simulink model "test"  (R2021b)
settings: Solver=FixedStepDiscrete  StartTime=0.0  StopTime=0.2  FixedStep=1e-6  RelTol=1e-3
InitFcn:
  | init_fcn
values from neighbouring files (symbols this model uses):
  Tint = 1e-6    (= 1e-06)    [init_fcn.m]
libraries: spsIGBTDiodeLib x6, spsVoltageMeasurementLib x4, spsSeriesRLCBranchLib x4, spsCurrentMeasurementLib x3, simulink x1, spsThreePhaseSourceLib x1, spspowerguiLib x1
settings Model: Creator=david  LastModifiedBy=david

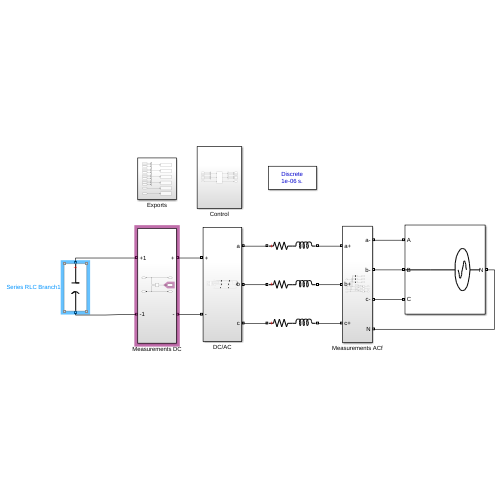
[thumbnail: Simulink's stored preview of the top-level diagram]
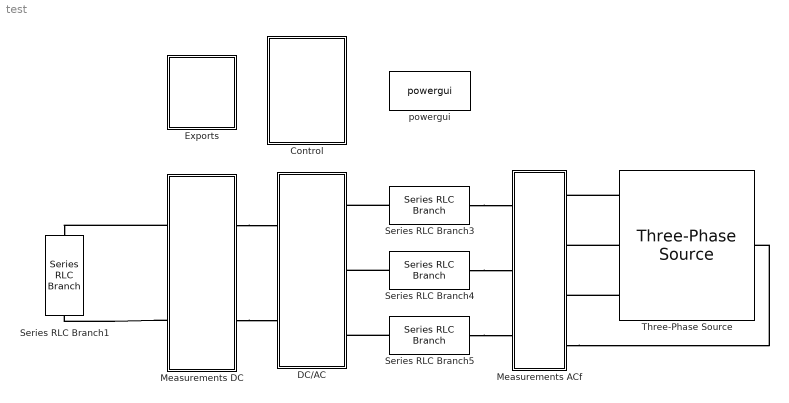
== system test ==
  Control : Subsystem
  DC/AC : Subsystem
  Exports : Subsystem
  Measurements ACf : Subsystem
  Measurements DC : Subsystem
  Series RLC Branch1 : spsSeriesRLCBranchLib/Series RLC Branch  LConnTagsString=__new0  RConnTagsString=__new0  BranchType=C  Resistance=0.2  Inductance=5e-3  SetiL0=off  InitialCurrent=0  Capacitance=3300e-6  Setx0=on  InitialVoltage=560  Measurements=None
  Series RLC Branch3 : spsSeriesRLCBranchLib/Series RLC Branch  LConnTagsString=__new0  RConnTagsString=__new0  BranchType=RL  Resistance=0.2  Inductance=5e-3  SetiL0=off  InitialCurrent=0  Capacitance=0  Setx0=off  InitialVoltage=0  Measurements=None
  Series RLC Branch4 : spsSeriesRLCBranchLib/Series RLC Branch  LConnTagsString=__new0  RConnTagsString=__new0  BranchType=RL  Resistance=0.2  Inductance=5e-3  SetiL0=off  InitialCurrent=0  Capacitance=0  Setx0=off  InitialVoltage=0  Measurements=None
  Series RLC Branch5 : spsSeriesRLCBranchLib/Series RLC Branch  LConnTagsString=__new0  RConnTagsString=__new0  BranchType=RL  Resistance=0.2  Inductance=5e-3  SetiL0=off  InitialCurrent=0  Capacitance=0  Setx0=off  InitialVoltage=0  Measurements=None
  Three-Phase Source : spsThreePhaseSourceLib/Three-Phase Source  InternalConnection=Yn  VoltagePhases=off  Voltage=400  PhaseAngle=0  Voltage_phases=[25e3 25e3 25e3]/sqrt(3)  PhaseAngles_phases=[0 -120 +120]  Frequency=50  NonIdealSource=on  SpecifyImpedance=off  Resistance=0  Inductance=0  ShortCircuitLevel=100e6  BaseVoltage=400  XRratio=7  BusType=swing  Pref=10e3  Qref=0  Prefabc=[10e3, 10e3, 10e3]  Qrefabc=[0, 0, 0]  Qmin=-inf  Qmax=inf
  powergui : spspowerguiLib/powergui  Priority=1  SimulationMode=Discrete  SampleTime=Tint  frequency=60  Iterations=50  frequencyindice=0  Pbase=100e6  ErrMax=1e-4  UnitsV=kV  UnitsW=MW  buscounter=0  FunctionMessages=off  echomessages=off  EnableUseOfTLC=off  CurrentSourceSwitches=off  DisableSnubberDevices=off  DisableRonSwitches=off  DisableVfSwitches=off  DisplayEquations=off  AutomaticDiscreteSolvers=off  SolverType=Tustin/Backward Euler (TBE)  Interpol=off  ExternalGateDelay=off  methode=off  Ts=100  x0status=blocks  SPID=on  SwTol=0  HookPort=off  NonlinearTolerance=1e-4  nMaxIteration=100  ContinueOnMaxIteration=off  RestoreLinks=warning  ResistiveCurrentMeasurement=off  Frange=[0:2:500]  Ylog=off  Xlog=on  ShowGrid=off  save=off  variable=ZData  structure=0  ZoomFFT=off  StartTime=0.0  cycles=1  DisplayStyle=1  fundamental=60  FreqAxis=off  MaxFrequency=1000  frequencyindicesteady=1  RmsSteady=1  display=off
  connections:
  Series RLC Branch3/LConn1 -- DC/AC/RConn1
  Measurements DC/LConn2 -- Series RLC Branch1/RConn1
  Measurements DC/LConn1 -- Series RLC Branch1/LConn1
  Measurements DC/RConn1 -- DC/AC/LConn1
  Measurements DC/RConn2 -- DC/AC/LConn2
  Series RLC Branch5/LConn1 -- DC/AC/RConn3
  Series RLC Branch4/LConn1 -- DC/AC/RConn2
  Three-Phase Source/RConn1 -- Measurements ACf/RConn1
  Three-Phase Source/RConn2 -- Measurements ACf/RConn2
  Three-Phase Source/RConn3 -- Measurements ACf/RConn3
  Series RLC Branch3/RConn1 -- Measurements ACf/LConn1
  Series RLC Branch5/RConn1 -- Measurements ACf/LConn3
  Series RLC Branch4/RConn1 -- Measurements ACf/LConn2
  Measurements ACf/RConn4 -- Three-Phase Source/LConn1

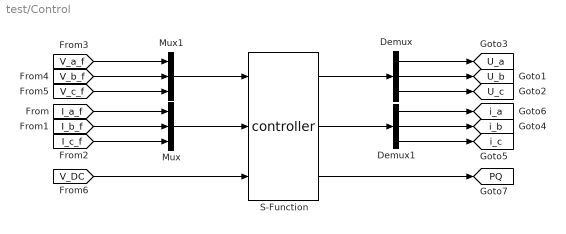
== system test/Control ==
  Demux : Demux  Outputs=3
  Demux1 : Demux  Outputs=3
  Mux : Mux  Inputs=3
  Mux1 : Mux  Inputs=3
  S-Function : S-Function  FunctionName=controller  SFunctionDeploymentMode=off  EnableBusSupport=off
  tag scope: PQ=global, U_a=global, U_b=global, U_c=global, i_a=global, i_b=global, i_c=global
  wires:
  [I_a_f] -> Mux/1
  [I_c_f] -> Mux/3
  Mux1/1 -> S-Function/1
  [V_a_f] -> Mux1/1
  [V_c_f] -> Mux1/3
  [I_b_f] -> Mux/2
  [V_b_f] -> Mux1/2
  Mux/1 -> S-Function/2
  S-Function/1 -> Demux/1
  S-Function/2 -> Demux1/1
  Demux/1 -> [U_a]
  Demux/2 -> [U_b]
  Demux/3 -> [U_c]
  Demux1/1 -> [i_a]
  Demux1/2 -> [i_b]
  Demux1/3 -> [i_c]
  S-Function/3 -> [PQ]
  [V_DC] -> S-Function/3

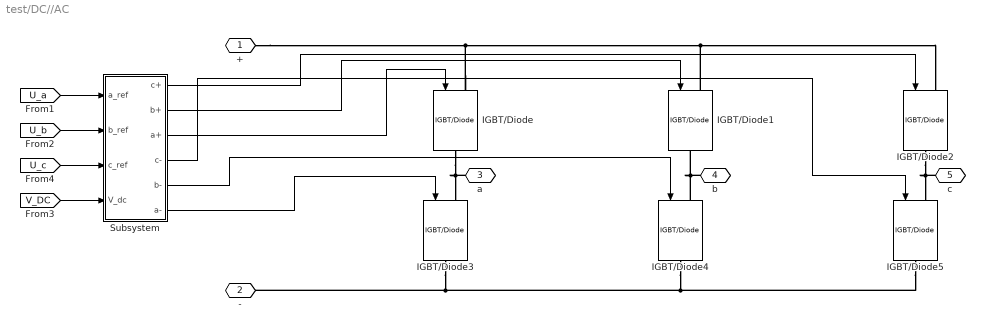
== system test/DC//AC ==
  IGBT/Diode{,1..5} (6 alike) : spsIGBTDiodeLib/IGBT//Diode  Ron=1e-3  Rs=1e5  Cs=inf  Measurements=off
  Subsystem : Subsystem
  + : PMIOPort  Side=Left
  - : PMIOPort  Port=2  Side=Left
  a : PMIOPort  Port=3  Side=Right
  b : PMIOPort  Port=4  Side=Right
  c : PMIOPort  Port=5  Side=Right
  wires:
  Subsystem/3(a+) -> IGBT/Diode/1
  Subsystem/2(b+) -> IGBT/Diode1/1
  Subsystem/5(b-) -> IGBT/Diode4/1
  Subsystem/1(c+) -> IGBT/Diode2/1
  Subsystem/4(c-) -> IGBT/Diode5/1
  [V_DC] -> Subsystem/4(V_dc)
  Subsystem/6(a-) -> IGBT/Diode3/1
  [U_b] -> Subsystem/2(b_ref)
  [U_c] -> Subsystem/3(c_ref)
  [U_a] -> Subsystem/1(a_ref)
  connections:
  IGBT/Diode2/RConn1 -- c/RConn1 -- IGBT/Diode5/LConn1
  IGBT/Diode/RConn1 -- a/RConn1 -- IGBT/Diode3/LConn1
  IGBT/Diode4/LConn1 -- b/RConn1 -- IGBT/Diode1/RConn1
  IGBT/Diode5/RConn1 -- IGBT/Diode4/RConn1 -- IGBT/Diode3/RConn1 -- -/RConn1
  IGBT/Diode/LConn1 -- IGBT/Diode2/LConn1 -- IGBT/Diode1/LConn1 -- +/RConn1

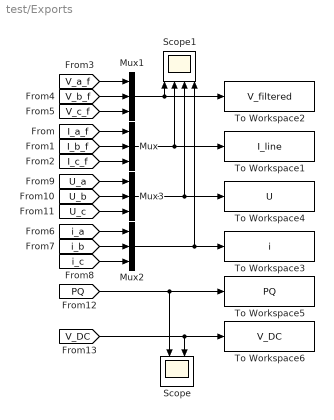
== system test/Exports ==
  Mux{,1..3} (4 alike) : Mux  Inputs=3
  Scope : Scope  NumInputPorts=2
  Scope1 : Scope  NumInputPorts=4
  To Workspace1 : ToWorkspace  VariableName=I_line  SaveFormat=Structure With Time  SampleTime=-1
  To Workspace2 : ToWorkspace  VariableName=V_filtered  SaveFormat=Structure With Time  SampleTime=-1
  To Workspace3 : ToWorkspace  VariableName=i  SaveFormat=Structure With Time  SampleTime=-1
  To Workspace4 : ToWorkspace  VariableName=U  SaveFormat=Structure With Time  SampleTime=-1
  To Workspace5 : ToWorkspace  VariableName=PQ  SaveFormat=Structure With Time  SampleTime=-1
  To Workspace6 : ToWorkspace  VariableName=V_DC  SaveFormat=Structure With Time  SampleTime=-1
  wires:
  [I_c_f] -> Mux/3
  [V_a_f] -> Mux1/1
  [I_a_f] -> Mux/1
  [I_b_f] -> Mux/2
  [V_b_f] -> Mux1/2
  [V_c_f] -> Mux1/3
  Mux1/1 -> Scope1/1, To Workspace2/1
  Mux/1 -> Scope1/2, To Workspace1/1
  [U_a] -> Mux3/1
  [U_c] -> Mux3/3
  [U_b] -> Mux3/2
  [i_a] -> Mux2/1
  [i_c] -> Mux2/3
  Mux3/1 -> Scope1/3, To Workspace4/1
  Mux2/1 -> Scope1/4, To Workspace3/1
  [i_b] -> Mux2/2
  [V_DC] -> Scope/2, To Workspace6/1
  [PQ] -> Scope/1, To Workspace5/1

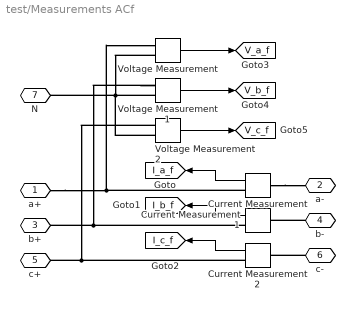
== system test/Measurements ACf ==
  Current Measurement : spsCurrentMeasurementLib/Current Measurement  PhasorSimulation=off  OutputType=Complex  PSBequivalent=0
  Current Measurement1 : spsCurrentMeasurementLib/Current Measurement  PhasorSimulation=off  OutputType=Complex  PSBequivalent=0
  Current Measurement2 : spsCurrentMeasurementLib/Current Measurement  PhasorSimulation=off  OutputType=Complex  PSBequivalent=0
  Voltage Measurement : spsVoltageMeasurementLib/Voltage Measurement  PhasorSimulation=off  OutputType=Complex  PSBequivalent=0
  Voltage Measurement1 : spsVoltageMeasurementLib/Voltage Measurement  PhasorSimulation=off  OutputType=Complex  PSBequivalent=0
  Voltage Measurement2 : spsVoltageMeasurementLib/Voltage Measurement  PhasorSimulation=off  OutputType=Complex  PSBequivalent=0
  a+ : PMIOPort  Side=Left
  a- : PMIOPort  Port=2  Side=Right
  b+ : PMIOPort  Port=3  Side=Left
  b- : PMIOPort  Port=4  Side=Right
  c+ : PMIOPort  Port=5  Side=Left
  c- : PMIOPort  Port=6  Side=Right
  N : PMIOPort  Port=7  Side=Right
  tag scope: I_a_f=global, I_b_f=global, I_c_f=global, V_a_f=global, V_b_f=global, V_c_f=global
  wires:
  Current Measurement1/1 -> [I_b_f]
  Voltage Measurement1/1 -> [V_b_f]
  Voltage Measurement/1 -> [V_a_f]
  Voltage Measurement2/1 -> [V_c_f]
  Current Measurement/1 -> [I_a_f]
  Current Measurement2/1 -> [I_c_f]
  connections:
  Voltage Measurement1/LConn1 -- Current Measurement1/RConn1 -- b+/RConn1
  Voltage Measurement2/LConn2 -- Voltage Measurement/LConn2 -- N/RConn1 -- Voltage Measurement1/LConn2
  Voltage Measurement2/LConn1 -- Current Measurement2/RConn1 -- c+/RConn1
  a+/RConn1 -- Current Measurement/RConn1 -- Voltage Measurement/LConn1
  Current Measurement/LConn1 -- a-/RConn1
  b-/RConn1 -- Current Measurement1/LConn1
  c-/RConn1 -- Current Measurement2/LConn1

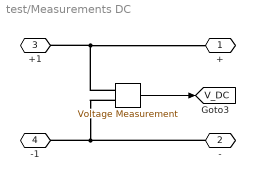
== system test/Measurements DC ==
  "  " : spsVoltageMeasurementLib/Voltage Measurement  PhasorSimulation=off  OutputType=Complex  PSBequivalent=0
  + : PMIOPort  Side=Right
  - : PMIOPort  Port=2  Side=Right
  +1 : PMIOPort  Port=3  Side=Left
  -1 : PMIOPort  Port=4  Side=Left
  tag scope: V_DC=global
  wires:
  "  "/1 -> [V_DC]
  connections:
  "  "/LConn1 -- +/RConn1 -- +1/RConn1
  -/RConn1 -- "  "/LConn2 -- -1/RConn1

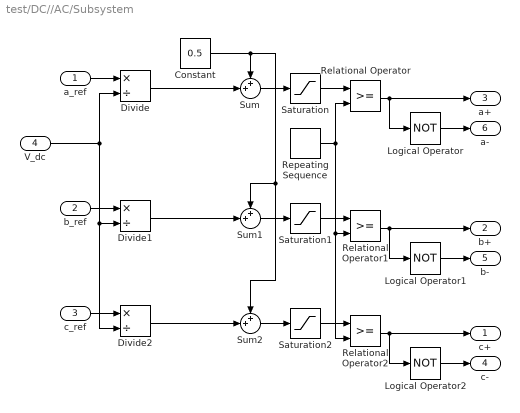
== system test/DC//AC/Subsystem ==
  a_ref : Inport
  b_ref : Inport  Port=2
  c_ref : Inport  Port=3
  V_dc : Inport  Port=4
  Constant : Constant  Value=0.5
  Divide : Product  Inputs=*/
  Divide1 : Product  Inputs=*/
  Divide2 : Product  Inputs=*/
  Logical Operator : Logic  Operator=NOT  AllPortsSameDT=off  OutDataTypeStr=boolean
  Logical Operator1 : Logic  Operator=NOT  AllPortsSameDT=off  OutDataTypeStr=boolean
  Logical Operator2 : Logic  Operator=NOT  AllPortsSameDT=off  OutDataTypeStr=boolean
  Relational Operator : RelationalOperator  OutDataTypeStr=boolean  RndMeth=Simplest
  Relational Operator1 : RelationalOperator  OutDataTypeStr=boolean  RndMeth=Simplest
  Relational Operator2 : RelationalOperator  OutDataTypeStr=boolean  RndMeth=Simplest
  Repeating Sequence : simulink/Sources/Repeating Sequence  rep_seq_t=[0 1/20000 1/10000]  rep_seq_y=[0 1 0]
  Saturation : Saturate  UpperLimit=1  LowerLimit=0
  Saturation1 : Saturate  UpperLimit=1  LowerLimit=0
  Saturation2 : Saturate  UpperLimit=1  LowerLimit=0
  Sum : Sum  Inputs=++|
  Sum1 : Sum  Inputs=++|
  Sum2 : Sum  Inputs=++|
  c+ : Outport
  b+ : Outport  Port=2
  a+ : Outport  Port=3
  c- : Outport  Port=4
  b- : Outport  Port=5
  a- : Outport  Port=6
  wires:
  a_ref/1 -> Divide/1
  Logical Operator/1 -> a-/1
  Divide/1 -> Sum/2
  Sum/1 -> Saturation/1
  Saturation/1 -> Relational Operator/1
  Relational Operator/1 -> a+/1, Logical Operator/1
  Saturation1/1 -> Relational Operator1/1
  Repeating Sequence/1 -> Relational Operator/2, Relational Operator2/2, Relational Operator1/2
  Divide1/1 -> Sum1/2
  Relational Operator1/1 -> b+/1, Logical Operator1/1
  b_ref/1 -> Divide1/1
  Logical Operator1/1 -> b-/1
  Sum1/1 -> Saturation1/1
  Sum2/1 -> Saturation2/1
  Divide2/1 -> Sum2/2
  Logical Operator2/1 -> c-/1
  Constant/1 -> Sum/1, Sum1/1, Sum2/1
  Saturation2/1 -> Relational Operator2/1
  Relational Operator2/1 -> c+/1, Logical Operator2/1
  c_ref/1 -> Divide2/1
  V_dc/1 -> Divide/2, Divide2/2, Divide1/2
